simulink model "main_sim"  (R2017b)
settings: Solver=FixedStepAuto  StartTime=0.0  StopTime=tmax  RelTol=1e-3
undefined symbols (not defined in the file): Bm, f_pwm, Jm, Km, Lm, Rm, ts, Vin_pwm, Vout_pwm
libraries: simulink x2
settings Model: Creator=JesusC  LastModifiedBy=JesusC

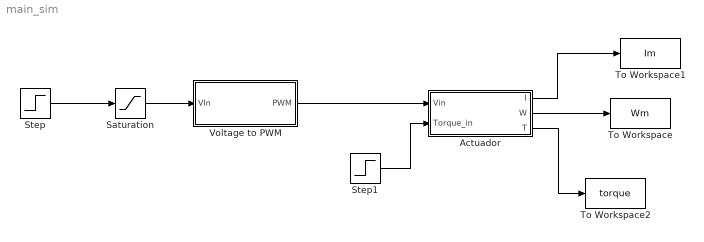
== system main_sim ==
  "Actuador " : Subsystem
  Saturation : Saturate  UpperLimit=Vin_pwm  LowerLimit=-Vin_pwm
  Step : Step  Time=0  After=0.8  SampleTime=0
  Step1 : Step  Time=0  After=0  SampleTime=0
  To Workspace : ToWorkspace  VariableName=Wm  SampleTime=ts
      settings: MaxDataPoints=N
  To Workspace1 : ToWorkspace  VariableName=Im  SampleTime=ts
      settings: MaxDataPoints=N
  To Workspace2 : ToWorkspace  VariableName=torque  SampleTime=ts
      settings: MaxDataPoints=N
  Voltage to PWM : Subsystem
  wires:
  Voltage to PWM/1(PWM) -> "Actuador "/1(Vin)
  "Actuador "/2(W) -> To Workspace/1
  Step1/1 -> "Actuador "/2(Torque_in)
  Saturation/1 -> Voltage to PWM/1(VIn)
  Step/1 -> Saturation/1
  "Actuador "/1(I) -> To Workspace1/1
  "Actuador "/3(T) -> To Workspace2/1

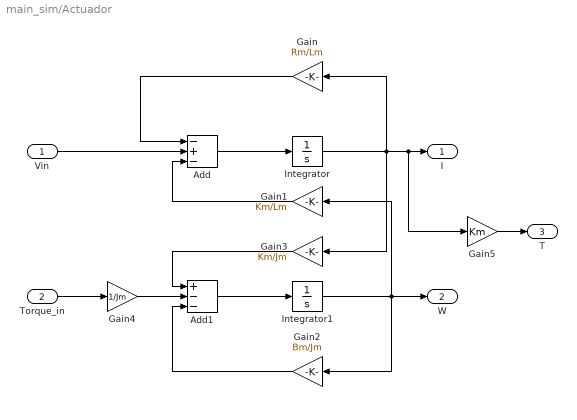
== system main_sim/Actuador  ==
  Vin : Inport
  Torque_in : Inport  Port=2
  Add : Sum  Inputs=-+-
  Add1 : Sum  Inputs=+--
  Gain : Gain  Gain=Rm/Lm
  Gain1 : Gain  Gain=Km/Lm
  Gain2 : Gain  Gain=Bm/Jm
  Gain3 : Gain  Gain=Km/Jm
  Gain4 : Gain  Gain=1/Jm
  Gain5 : Gain  Gain=Km
  Integrator : Integrator
  Integrator1 : Integrator
  I : Outport
  W : Outport  Port=2
  T : Outport  Port=3
  wires:
  Vin/1 -> Add/2
  Integrator/1 -> Gain3/1, Gain/1, Gain5/1, I/1
  Gain/1 -> Add/1
  Integrator1/1 -> Gain2/1, Gain1/1, W/1
  Gain1/1 -> Add/3
  Add/1 -> Integrator/1
  Add1/1 -> Integrator1/1
  Gain2/1 -> Add1/3
  Gain3/1 -> Add1/1
  Torque_in/1 -> Gain4/1
  Gain4/1 -> Add1/2
  Gain5/1 -> T/1

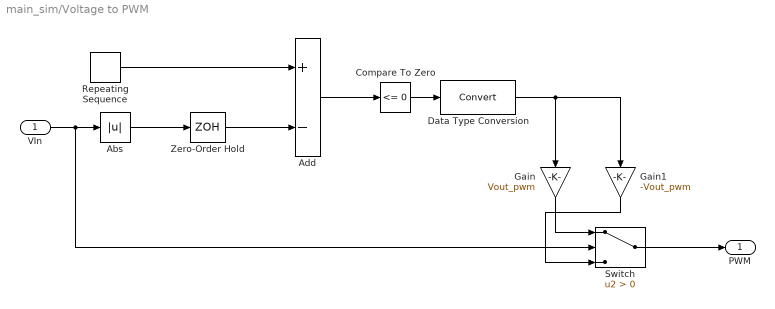
== system main_sim/Voltage to PWM ==
  VIn : Inport
  Abs : Abs
  Add : Sum  Inputs=+-
  Compare To Zero : simulink/Logic and Bit Operations/Compare To Zero  relop=<=  OutDataTypeStr=boolean
  Data Type Conversion : DataTypeConversion
  Gain : Gain  Gain=Vout_pwm
  Gain1 : Gain  Gain=-Vout_pwm
  Repeating Sequence : simulink/Sources/Repeating Sequence  rep_seq_t=[0 1/f_pwm]  rep_seq_y=[0 Vin_pwm]
  Switch : Switch  Criteria=u2 > Threshold
  Zero-Order Hold : ZeroOrderHold  SampleTime=-1
  PWM : Outport
  wires:
  Repeating Sequence/1 -> Add/1
  Add/1 -> Compare To Zero/1
  Zero-Order Hold/1 -> Add/2
  Abs/1 -> Zero-Order Hold/1
  VIn/1 -> Switch/2, Abs/1
  Gain/1 -> Switch/1
  Gain1/1 -> Switch/3
  Compare To Zero/1 -> Data Type Conversion/1
  Switch/1 -> PWM/1
  Data Type Conversion/1 -> Gain/1, Gain1/1
